simulink model "ed4"  (R2024a)
settings: Solver=VariableStepAuto  StartTime=0.0  StopTime=0.10  RelTol=1e-3
libraries: spsIGBTLib x6, spsDCVoltageSourceLib x1, spsPermanentMagnetSynchronousMachineLib x1, spsVoltageMeasurementLib x1, sps_lib x1
settings SolverCC: ZeroCrossAlgorithm=Adaptive
settings DebuggingCC: MaskedZcDiagnostic=none  IgnoredZcDiagnostic=none
settings RTWCC: GPUComputeCapability=3.5

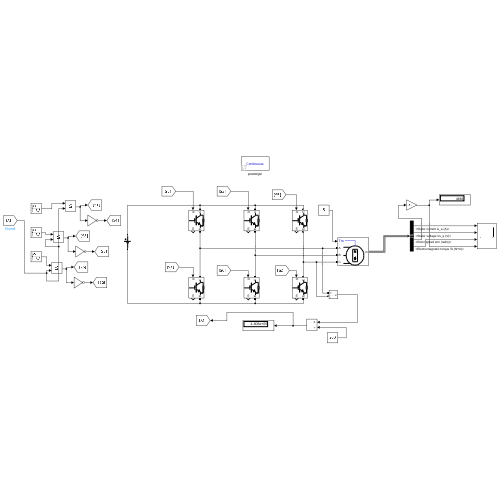
[thumbnail: Simulink's stored preview of the top-level diagram]
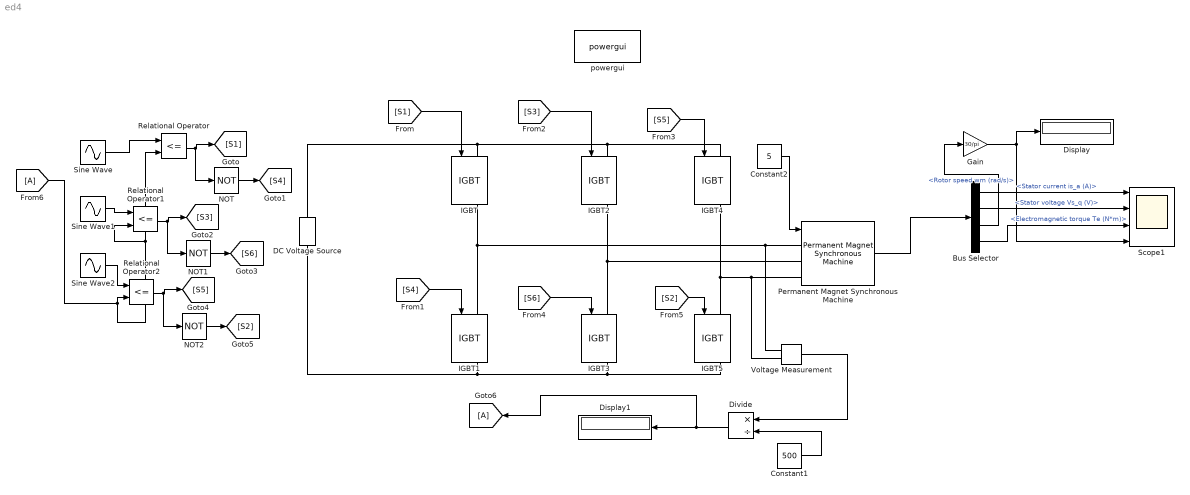
== system ed4 ==
  Bus Selector : BusSelector  OutputSignals=Stator current is_a (A),Stator voltage Vs_q (V),Rotor speed wm (rad/s),Electromagnetic torque Te (N*m)
  Constant1 : Constant  Value=500
  Constant2 : Constant  Value=5
  DC Voltage Source : spsDCVoltageSourceLib/DC Voltage Source  Amplitude=400  Measurements=Voltage
  Display : Display
  Display1 : Display
  Divide : Product  Inputs=*/  RndMeth=Zero  SaturateOnIntegerOverflow=on
  From6 : From
  Gain : Gain  Gain=30/pi
  Goto6 : Goto
  IGBT{,1..5} (6 alike) : spsIGBTLib/IGBT  Ron=0.001  Lon=0  Vf=1  Tf=1e-6  Tt=2e-6  IC=0  Rs=1e5  Cs=inf  Measurements=on
  NOT : Logic  Operator=NOT  IconShape=distinctive  AllPortsSameDT=off  OutDataTypeStr=boolean
  NOT1 : Logic  Operator=NOT  IconShape=distinctive  AllPortsSameDT=off  OutDataTypeStr=boolean
  NOT2 : Logic  Operator=NOT  IconShape=distinctive  AllPortsSameDT=off  OutDataTypeStr=boolean
  Permanent Magnet Synchronous Machine : spsPermanentMagnetSynchronousMachineLib/Permanent Magnet Synchronous Machine  NbPhases=3  FluxDistribution=Sinusoidal  RotorType=Round  MechanicalLoad=Torque Tm  PresetModel=No  ShowDetailedParameters=on  MeasurementBus=off  Resistance=0.0485  Inductance=8.5e-3  dqInductances=[8.5e-3,8.5e-3]  La=0.000395  MachineConstant=Flux linkage established by magnets (V.s)  Flux=0.1194  VoltageCst=86.6271  TorqueCst=0.7164  Flat=120  Mechanical=[0.0027 0.0004924 4 0]  PolePairs=4  InitialConditions=[0,0, 0,0]  InitialConditions5ph=[0 0 0 0 0 0]  RefAngle=90 degrees behind phase A axis (modified Park)  IterativeDiscreteModel=Trapezoidal non iterative  TsBlock=-1  TsPowergui=0
  Relational Operator : RelationalOperator  Operator=<=  OutDataTypeStr=boolean  RndMeth=Simplest  InputSameDT=off
  Relational Operator1 : RelationalOperator  Operator=<=  OutDataTypeStr=boolean  RndMeth=Simplest  InputSameDT=off
  Relational Operator2 : RelationalOperator  Operator=<=  OutDataTypeStr=boolean  RndMeth=Simplest  InputSameDT=off
  Scope1 : Scope  NumInputPorts=4
  Sine Wave : Sin  Frequency=50*2*pi  SampleTime=0
  Sine Wave1 : Sin  Frequency=50*2*pi  Phase=120*(pi/180)  SampleTime=0
  Sine Wave2 : Sin  Frequency=50*2*pi  Phase=240*(pi/180)  SampleTime=0
  Voltage Measurement : spsVoltageMeasurementLib/Voltage Measurement  PhasorSimulation=off  OutputType=Complex  PSBequivalent=0
  powergui : sps_lib/powergui  Priority=1  SimulationMode=Continuous  SampleTime=50e-6  frequency=60  Iterations=50  frequencyindice=0  Pbase=100e6  ErrMax=1e-4  UnitsV=kV  UnitsW=MW  buscounter=0  FunctionMessages=off  echomessages=off  EnableUseOfTLC=off  CurrentSourceSwitches=off  DisableSnubberDevices=off  DisableRonSwitches=off  DisableVfSwitches=off  DisplayEquations=off  AutomaticDiscreteSolvers=off  SolverType=Tustin/Backward Euler (TBE)  Interpol=off  ExternalGateDelay=off  methode=off  Ts=100  x0status=blocks  SPID=on  SwTol=0  HookPort=off  NonlinearTolerance=1e-4  nMaxIteration=100  ContinueOnMaxIteration=off  RestoreLinks=warning  ResistiveCurrentMeasurement=off  Frange=[0:2:500]  Ylog=off  Xlog=on  ShowGrid=off  save=off  variable=ZData  structure=0  ZoomFFT=off  StartTime=0.0  cycles=1  DisplayStyle=1  fundamental=60  FreqAxis=off  MaxFrequency=1000  frequencyindicesteady=1  RmsSteady=1  display=off
  wires:
  Permanent Magnet Synchronous Machine/1 -> Bus Selector/1
  Sine Wave/1 -> Relational Operator/1
  From6/1 -> Relational Operator1/2, Relational Operator/2, Relational Operator2/2
  Relational Operator/1 -> NOT/1, [S1]
  NOT/1 -> [S4]
  [S1] -> IGBT/1
  [S4] -> IGBT1/1
  Relational Operator1/1 -> NOT1/1, [S3]
  NOT1/1 -> [S6]
  Sine Wave1/1 -> Relational Operator1/1
  Relational Operator2/1 -> NOT2/1, [S5]
  NOT2/1 -> [S2]
  Sine Wave2/1 -> Relational Operator2/1
  [S6] -> IGBT3/1
  [S3] -> IGBT2/1
  [S5] -> IGBT4/1
  [S2] -> IGBT5/1
  Gain/1 -> Scope1/4, Display/1
  Voltage Measurement/1 -> Divide/1
  Constant1/1 -> Divide/2
  Divide/1 -> Goto6/1, Display1/1
  Constant2/1 -> Permanent Magnet Synchronous Machine/1
  Bus Selector/1 -> Scope1/1  "<Stator current is_a (A)>"
  Bus Selector/4 -> Scope1/3  "<Electromagnetic torque Te (N*m)>"
  Bus Selector/3 -> Gain/1  "<Rotor speed wm (rad/s)>"
  Bus Selector/2 -> Scope1/2  "<Stator voltage Vs_q (V)>"
  connections:
  IGBT1/LConn1 -- Permanent Magnet Synchronous Machine/LConn1 -- Voltage Measurement/LConn1 -- IGBT/RConn1
  IGBT3/LConn1 -- IGBT2/RConn1 -- Permanent Magnet Synchronous Machine/LConn2
  IGBT5/LConn1 -- Permanent Magnet Synchronous Machine/LConn3 -- Voltage Measurement/LConn2 -- IGBT4/RConn1
  DC Voltage Source/RConn1 -- IGBT4/LConn1 -- IGBT2/LConn1 -- IGBT/LConn1
  IGBT5/RConn1 -- DC Voltage Source/LConn1 -- IGBT1/RConn1 -- IGBT3/RConn1
